simulink model "PMSM_FOC_Encoder_ST"  (R2013b)
settings: Solver=FixedStepDiscrete  StartTime=0.0  StopTime=0.8  FixedStep=1/10000  RelTol=1e-3
PostLoadFcn:
  | PMSM_Params
undefined symbols (not defined in the file or in its folder): Params, PC10, PC11, uart4, usart3
libraries: ADC_Lib x5, GPIO_Lib x5, TIMERS_Lib x2, USART_Lib x1
settings Model: Creator=Alex  LastModifiedBy=reynaudp
settings OptimizationCC: ExpressionDepthLimit=2147483647  OptimizeModelRefInitCode=on  LifeSpan=1
settings DebuggingCC: StateNameClashWarn=warning
settings HardwareCC: ProdLargestAtomicInteger=Integer  ProdLargestAtomicFloat=Float  ProdIntDivRoundTo=Zero  ProdEndianess=LittleEndian  ProdHWDeviceType=STMicroelectronics->STM32F4xx 32-bit Cortex-M4  TargetLargestAtomicInteger=Integer  TargetLargestAtomicFloat=Float  TargetIntDivRoundTo=Zero  TargetEndianess=LittleEndian  TargetHWDeviceType=STMicroelectronics->STM32F4xx 32-bit Cortex-M4
settings RTWCC: SystemTargetFile=stm32F4xx.tlc  TemplateMakefile=stm32F4xx.tmf  Description=stm32F4xx (Embedded Target)  GenerateReport=on  ProcessScript=stm32F4xx_make_rtw_hook  IncludeHyperlinkInReport=on  LaunchReport=on  GenerateCodeReplacementReport=on
settings CodeAppCC: IgnoreCustomStorageClasses=off  MaxIdLength=64  CustomSymbolStrType=$N$R$M  InternalIdentifier=Classic
settings STFCustomTargetCC: ParMdlRefBuildCompliant=on  IncludeMdlTerminateFcn=off  CombineOutputUpdateFcns=on  ERTCustomFileBanners=on  SupportContinuousTime=off  SupportNonInlinedSFcns=off  MATLABClassNameForMDSCustomization=Simulink.SoftwareTarget.ERTCustomization  GRTInterface=off  SystemTargetFile=stm32F4xx.tlc
settings ERTTargetCC: CodeReplacementLibrary=ANSI_C  CompOptLevelCompliant=off  ConcurrentExecutionCompliant=off  IncludeMdlTerminateFcn=off  ERTFirstTimeCompliant=off  ModelStepFunctionPrototypeControlCompliant=off  CPPClassGenCompliant=off  InlinedParameterPlacement=NonHierarchical  ERTSrcFileBannerTemplate=sourceFileTemplate.cgt  ERTHdrFileBannerTemplate=sourceFileTemplate.cgt  ERTDataSrcFileTemplate=sourceFileTemplate.cgt  ERTDataHdrFileTemplate=sourceFileTemplate.cgt  ERTCustomFileTemplate=customRoutineProcess.tlc

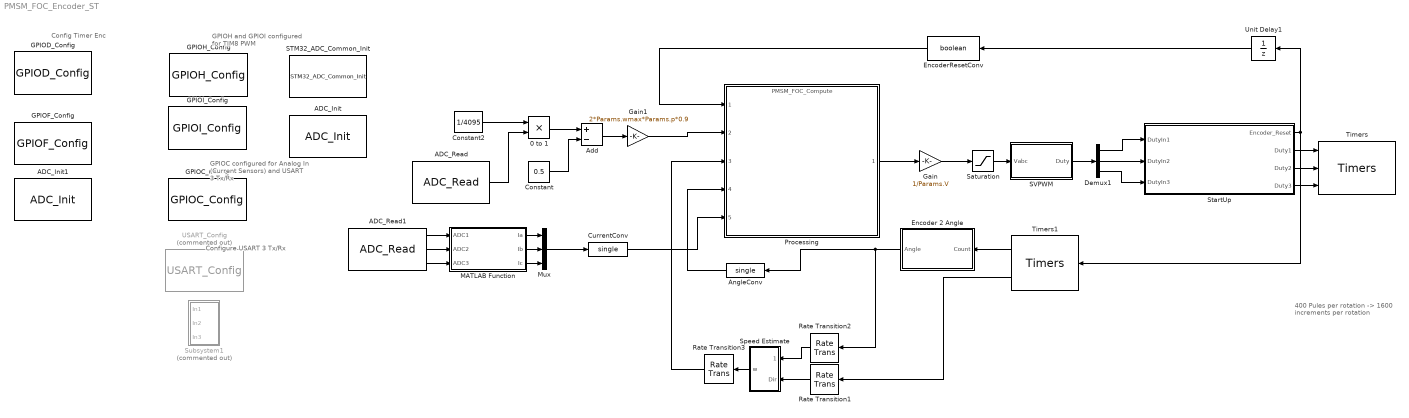
== system PMSM_FOC_Encoder_ST ==
  note: Config Timer Enc
  note: 400 Pules per rotation -> 1600 increments per rotation
  note: Configure USART 3 Tx/Rx
  note: GPIOC configured for Analog In (Current Sensors)
      | and  USART 3 Tx/Rx
  note: GPIOH and GPIOI configured for TIM8 PWM
  0 to 1 : Product  RndMeth=Zero
  ADC_Init : ADC_Lib/ADC_Init  ADC_Name=ADC1  ADC_Type=Regular  ADC_Default=off  ADC_Offset=0  ADC_Resolution=ADC_Resolution_12b  ADC_ScanConvMode=Multichannels  ADC_ContinuousConvMode=on  ADC_ExtTrigPol=ADC_ExternalTrigConvEdge_Rising  ADC_ExtTrigInjPol=ADC_ExternalTrigInjecConvEdge_None  ADC_ExtTrig=ADC_ExternalTrigConv_T8_TRGO  ADC_ExtTrigInj=ADC_ExternalTrigInjecConv_T1_CC4  ADC_DataAlign=ADC_DataAlign_Right  ADC_NbConv=3  ADC_DMA_channel=DMA_Channel_0  ADC_DMA_stream=DMA2_Stream0  ADC_Watchdog_Enable=off  ADC_Watchdog_Command=ADC_AnalogWatchdog_None  ADC_Watchdog_NumChan=0  ADC_Watchdog_HighThreshold=4095  ADC_Watchdog_lowThreshold=0  ADC_Ch0=off  ADC_Ch0T=Regular  ADC_Ch0L=PA0  ADC_Ch1=off  ADC_Ch1T=Regular  ADC_Ch1L=PA1  ADC_Ch2=off  ADC_Ch2T=Regular  ADC_Ch2L=PA2  ADC_Ch3=off  ADC_Ch3T=Regular  ADC_Ch3L=PA3  ADC_Ch4=off  ADC_Ch4T=Regular  ADC_Ch4L=PA4  ADC_Ch5=off  ADC_Ch5T=Regular  ADC_Ch5L=PA5  ADC_Ch6=off  ADC_Ch6T=Regular  ADC_Ch6L=PA6  ADC_Ch7=off  ADC_Ch7T=Regular  ADC_Ch7L=PA7  ADC_Ch8=off  ADC_Ch8T=Regular  ADC_Ch8L=PB0  ADC_Ch9=off  ADC_Ch9T=Regular  ADC_Ch9L=PB1  ADC_Ch10=off  ADC_Ch10T=Regular  ADC_Ch10L=PC0  ADC_Ch11=on  ADC_Ch11T=Regular  ADC_Ch11L=PC1  ADC_Ch12=on  ADC_Ch12T=Regular  ADC_Ch12L=PC2  ADC_Ch13=on  ADC_Ch13T=Regular  ADC_Ch13L=PC3  ADC_Ch14=off  ADC_Ch14T=Regular  ADC_Ch14L=PC4  ADC_Ch15=off  ADC_Ch15T=Regular  ADC_Ch15L=PC5  ADC_Ch16=off  ADC_Ch16T=Regular  ADC_Ch16L=Temp.Sensor  ADC_Ch17=off  ADC_Ch17T=Regular  ADC_Ch17L=Vrefint  ADC_Ch18=off  ADC_Ch18T=Regular  ADC_Ch18L=Vbat
  ADC_Init1 : ADC_Lib/ADC_Init  ADC_Name=ADC3  ADC_Type=Regular  ADC_Default=off  ADC_Offset=0  ADC_Resolution=ADC_Resolution_12b  ADC_ScanConvMode=One_channel  ADC_ContinuousConvMode=on  ADC_ExtTrigPol=ADC_ExternalTrigConvEdge_None  ADC_ExtTrigInjPol=ADC_ExternalTrigInjecConvEdge_None  ADC_ExtTrig=ADC_ExternalTrigConv_T1_CC1  ADC_ExtTrigInj=ADC_ExternalTrigInjecConv_T1_CC4  ADC_DataAlign=ADC_DataAlign_Right  ADC_NbConv=1  ADC_DMA_channel=not_used  ADC_DMA_stream=not_used  ADC_Watchdog_Enable=off  ADC_Watchdog_Command=ADC_AnalogWatchdog_None  ADC_Watchdog_NumChan=0  ADC_Watchdog_HighThreshold=4095  ADC_Watchdog_lowThreshold=0  ADC_Ch0=off  ADC_Ch0T=Regular  ADC_Ch0L=PA0  ADC_Ch1=off  ADC_Ch1T=Regular  ADC_Ch1L=PA1  ADC_Ch2=off  ADC_Ch2T=Regular  ADC_Ch2L=PA2  ADC_Ch3=off  ADC_Ch3T=Regular  ADC_Ch3L=PA3  ADC_Ch4=off  ADC_Ch4T=Regular  ADC_Ch4L=PF6  ADC_Ch5=off  ADC_Ch5T=Regular  ADC_Ch5L=PF7  ADC_Ch6=off  ADC_Ch6T=Regular  ADC_Ch6L=PF8  ADC_Ch7=on  ADC_Ch7T=Regular  ADC_Ch7L=PF9  ADC_Ch8=off  ADC_Ch8T=Regular  ADC_Ch8L=PF10  ADC_Ch9=off  ADC_Ch9T=Regular  ADC_Ch9L=PF3  ADC_Ch10=off  ADC_Ch10T=Regular  ADC_Ch10L=PC0  ADC_Ch11=off  ADC_Ch11T=Regular  ADC_Ch11L=PC1  ADC_Ch12=off  ADC_Ch12T=Regular  ADC_Ch12L=PC2  ADC_Ch13=off  ADC_Ch13T=Regular  ADC_Ch13L=PC3  ADC_Ch14=off  ADC_Ch14T=Regular  ADC_Ch14L=PF4  ADC_Ch15=off  ADC_Ch15T=Regular  ADC_Ch15L=PF5  ADC_Ch16=off  ADC_Ch16T=Regular  ADC_Ch17=off  ADC_Ch17T=Regular  ADC_Ch18=off  ADC_Ch18T=Regular
  ADC_Read : ADC_Lib/ADC_Read  ADC_Name=ADC3  ADC_Ch0=off  ADC_Ch1=off  ADC_Ch2=off  ADC_Ch3=off  ADC_Ch4=off  ADC_Ch5=off  ADC_Ch6=off  ADC_Ch7=on  ADC_Ch8=off  ADC_Ch9=off  ADC_Ch10=off  ADC_Ch11=off  ADC_Ch12=off  ADC_Ch13=off  ADC_Ch14=off  ADC_Ch15=off  ADC_Ch16=off  ADC_Ch17=off  ADC_Ch18=off
  ADC_Read1 : ADC_Lib/ADC_Read  ADC_Name=ADC1  ADC_Ch0=off  ADC_Ch1=off  ADC_Ch2=off  ADC_Ch3=off  ADC_Ch4=off  ADC_Ch5=off  ADC_Ch6=off  ADC_Ch7=off  ADC_Ch8=off  ADC_Ch9=off  ADC_Ch10=off  ADC_Ch11=on  ADC_Ch12=on  ADC_Ch13=on  ADC_Ch14=off  ADC_Ch15=off  ADC_Ch16=off  ADC_Ch17=off  ADC_Ch18=off
  Add : Sum  Inputs=+-
  AngleConv : DataTypeConversion  OutDataTypeStr=single
  Constant : Constant  Value=0.5
  Constant2 : Constant  Value=1/4095
  CurrentConv : DataTypeConversion  OutDataTypeStr=single
  Demux1 : Demux  Outputs=3
  Encoder 2 Angle : MATLAB Function  TreatAsAtomicUnit=on
      settings: MinAlgLoopOccurrences=on
  EncoderResetConv : DataTypeConversion  OutDataTypeStr=boolean
  GPIOC_Config : GPIO_Lib/GPIOC_Config  Pin0_Use=off  Pin1_Use=on  Pin2_Use=on  Pin3_Use=on  Pin4_Use=off  Pin5_Use=off  Pin6_Use=off  Pin7_Use=on  Pin8_Use=off  Pin9_Use=off  Pin10_Use=on  Pin11_Use=on  Pin12_Use=off  Pin13_Use=off  Pin14_Use=off  Pin15_Use=off  Pin0_Speed=GPIO_Speed_2MHz  Pin1_Speed=GPIO_Speed_25MHz  Pin2_Speed=GPIO_Speed_25MHz  Pin3_Speed=GPIO_Speed_25MHz  Pin4_Speed=GPIO_Speed_2MHz  Pin5_Speed=GPIO_Speed_2MHz  Pin6_Speed=GPIO_Speed_2MHz  Pin7_Speed=GPIO_Speed_50MHz  Pin8_Speed=GPIO_Speed_2MHz  Pin9_Speed=GPIO_Speed_2MHz  Pin10_Speed=GPIO_Speed_2MHz  Pin11_Speed=GPIO_Speed_2MHz  Pin12_Speed=GPIO_Speed_2MHz  Pin13_Speed=GPIO_Speed_2MHz  Pin14_Speed=GPIO_Speed_2MHz  Pin15_Speed=GPIO_Speed_2MHz  Pin0_Mode=GPIO_Mode_OUT  Pin1_Mode=GPIO_Mode_AN  Pin2_Mode=GPIO_Mode_AN  Pin3_Mode=GPIO_Mode_AN  Pin4_Mode=GPIO_Mode_OUT  Pin5_Mode=GPIO_Mode_OUT  Pin6_Mode=GPIO_Mode_OUT  Pin7_Mode=GPIO_Mode_OUT  Pin8_Mode=GPIO_Mode_OUT  Pin9_Mode=GPIO_Mode_OUT  Pin10_Mode=GPIO_Mode_AF  Pin11_Mode=GPIO_Mode_AF  Pin12_Mode=GPIO_Mode_OUT  Pin13_Mode=GPIO_Mode_OUT  Pin14_Mode=GPIO_Mode_OUT  Pin15_Mode=GPIO_Mode_OUT  Pin0_Type=GPIO_OType_PP  Pin1_Type=GPIO_OType_PP  Pin2_Type=GPIO_OType_PP  Pin3_Type=GPIO_OType_PP  Pin4_Type=GPIO_OType_PP  Pin5_Type=GPIO_OType_PP  Pin6_Type=GPIO_OType_PP  Pin7_Type=GPIO_OType_PP  Pin8_Type=GPIO_OType_PP  Pin9_Type=GPIO_OType_PP  Pin10_Type=GPIO_OType_PP  Pin11_Type=GPIO_OType_PP  Pin12_Type=GPIO_OType_PP  Pin13_Type=GPIO_OType_PP  Pin14_Type=GPIO_OType_PP  Pin15_Type=GPIO_OType_PP  Pin0_PuPd=GPIO_PuPd_NOPULL  Pin1_PuPd=GPIO_PuPd_NOPULL  Pin2_PuPd=GPIO_PuPd_NOPULL  Pin3_PuPd=GPIO_PuPd_NOPULL  Pin4_PuPd=GPIO_PuPd_NOPULL  Pin5_PuPd=GPIO_PuPd_NOPULL  Pin6_PuPd=GPIO_PuPd_NOPULL  Pin7_PuPd=GPIO_PuPd_NOPULL  Pin8_PuPd=GPIO_PuPd_NOPULL  Pin9_PuPd=GPIO_PuPd_NOPULL  Pin10_PuPd=GPIO_PuPd_NOPULL  Pin11_PuPd=GPIO_PuPd_NOPULL  Pin12_PuPd=GPIO_PuPd_NOPULL  Pin13_PuPd=GPIO_PuPd_NOPULL  Pin14_PuPd=GPIO_PuPd_NOPULL  Pin15_PuPd=GPIO_PuPd_NOPULL  Pin0_AF=GPIO_AF_OTG_HS  Pin1_AF=GPIO_AF_ETH  Pin2_AF=GPIO_AF_SPI2  Pin3_AF=GPIO_AF_SPI2  Pin4_AF=GPIO_AF_ETH  Pin5_AF=GPIO_AF_EVENTOUT  Pin6_AF=GPIO_AF_TIM3  Pin7_AF=GPIO_AF_TIM3  Pin8_AF=GPIO_AF_TIM3  Pin9_AF=GPIO_AF_MCO  Pin10_AF=GPIO_AF_USART3  Pin11_AF=GPIO_AF_USART3  Pin12_AF=GPIO_AF_USART3  Pin0_Set=off  Pin1_Set=off  Pin2_Set=off  Pin3_Set=off  Pin4_Set=off  Pin5_Set=off  Pin6_Set=off  Pin7_Set=off  Pin8_Set=off  Pin9_Set=off  Pin10_Set=off  Pin11_Set=off  Pin12_Set=off  Pin13_Set=off  Pin14_Set=off  Pin15_Set=off
  GPIOD_Config : GPIO_Lib/GPIOD_Config  Pin0_Use=off  Pin1_Use=off  Pin2_Use=off  Pin3_Use=off  Pin4_Use=off  Pin5_Use=off  Pin6_Use=off  Pin7_Use=off  Pin8_Use=off  Pin9_Use=off  Pin10_Use=off  Pin11_Use=off  Pin12_Use=on  Pin13_Use=on  Pin14_Use=off  Pin15_Use=off  Pin0_Speed=GPIO_Speed_2MHz  Pin1_Speed=GPIO_Speed_2MHz  Pin2_Speed=GPIO_Speed_2MHz  Pin3_Speed=GPIO_Speed_2MHz  Pin4_Speed=GPIO_Speed_2MHz  Pin5_Speed=GPIO_Speed_2MHz  Pin6_Speed=GPIO_Speed_2MHz  Pin7_Speed=GPIO_Speed_2MHz  Pin8_Speed=GPIO_Speed_2MHz  Pin9_Speed=GPIO_Speed_2MHz  Pin10_Speed=GPIO_Speed_2MHz  Pin11_Speed=GPIO_Speed_2MHz  Pin12_Speed=GPIO_Speed_50MHz  Pin13_Speed=GPIO_Speed_50MHz  Pin14_Speed=GPIO_Speed_2MHz  Pin15_Speed=GPIO_Speed_2MHz  Pin0_Mode=GPIO_Mode_OUT  Pin1_Mode=GPIO_Mode_OUT  Pin2_Mode=GPIO_Mode_OUT  Pin3_Mode=GPIO_Mode_OUT  Pin4_Mode=GPIO_Mode_OUT  Pin5_Mode=GPIO_Mode_OUT  Pin6_Mode=GPIO_Mode_OUT  Pin7_Mode=GPIO_Mode_OUT  Pin8_Mode=GPIO_Mode_OUT  Pin9_Mode=GPIO_Mode_OUT  Pin10_Mode=GPIO_Mode_OUT  Pin11_Mode=GPIO_Mode_OUT  Pin12_Mode=GPIO_Mode_AF  Pin13_Mode=GPIO_Mode_AF  Pin14_Mode=GPIO_Mode_OUT  Pin15_Mode=GPIO_Mode_OUT  Pin0_Type=GPIO_OType_PP  Pin1_Type=GPIO_OType_PP  Pin2_Type=GPIO_OType_PP  Pin3_Type=GPIO_OType_PP  Pin4_Type=GPIO_OType_PP  Pin5_Type=GPIO_OType_PP  Pin6_Type=GPIO_OType_PP  Pin7_Type=GPIO_OType_PP  Pin8_Type=GPIO_OType_PP  Pin9_Type=GPIO_OType_PP  Pin10_Type=GPIO_OType_PP  Pin11_Type=GPIO_OType_PP  Pin12_Type=GPIO_OType_PP  Pin13_Type=GPIO_OType_PP  Pin14_Type=GPIO_OType_PP  Pin15_Type=GPIO_OType_PP  Pin0_PuPd=GPIO_PuPd_NOPULL  Pin1_PuPd=GPIO_PuPd_NOPULL  Pin2_PuPd=GPIO_PuPd_NOPULL  Pin3_PuPd=GPIO_PuPd_NOPULL  Pin4_PuPd=GPIO_PuPd_NOPULL  Pin5_PuPd=GPIO_PuPd_NOPULL  Pin6_PuPd=GPIO_PuPd_NOPULL  Pin7_PuPd=GPIO_PuPd_NOPULL  Pin8_PuPd=GPIO_PuPd_NOPULL  Pin9_PuPd=GPIO_PuPd_NOPULL  Pin10_PuPd=GPIO_PuPd_NOPULL  Pin11_PuPd=GPIO_PuPd_NOPULL  Pin12_PuPd=GPIO_PuPd_NOPULL  Pin13_PuPd=GPIO_PuPd_NOPULL  Pin14_PuPd=GPIO_PuPd_NOPULL  Pin15_PuPd=GPIO_PuPd_NOPULL  Pin0_AF=GPIO_AF_CAN1  Pin1_AF=GPIO_AF_CAN1  Pin2_AF=GPIO_AF_TIM3  Pin3_AF=GPIO_AF_USART2  Pin4_AF=GPIO_AF_USART2  Pin5_AF=GPIO_AF_EVENTOUT  Pin6_AF=GPIO_AF_USART2  Pin7_AF=GPIO_AF_USART2  Pin8_AF=GPIO_AF_USART3  Pin9_AF=GPIO_AF_USART3  Pin10_AF=GPIO_AF_USART3  Pin11_AF=GPIO_AF_USART3  Pin12_AF=GPIO_AF_TIM4  Pin13_AF=GPIO_AF_TIM4  Pin14_AF=GPIO_AF_TIM4  Pin15_AF=GPIO_AF_EVENTOUT  Pin0_Set=off  Pin1_Set=off  Pin2_Set=off  Pin3_Set=off  Pin4_Set=off  Pin5_Set=off  Pin6_Set=off  Pin7_Set=off  Pin8_Set=off  Pin9_Set=off  Pin10_Set=off  Pin11_Set=off  Pin12_Set=off  Pin13_Set=off  Pin14_Set=off  Pin15_Set=off
  GPIOF_Config : GPIO_Lib/GPIOF_Config  Pin0_Use=off  Pin1_Use=off  Pin2_Use=off  Pin3_Use=off  Pin4_Use=off  Pin5_Use=off  Pin6_Use=off  Pin7_Use=off  Pin8_Use=off  Pin9_Use=on  Pin10_Use=off  Pin11_Use=off  Pin12_Use=off  Pin13_Use=off  Pin14_Use=off  Pin15_Use=off  Pin0_Speed=GPIO_Speed_2MHz  Pin1_Speed=GPIO_Speed_2MHz  Pin2_Speed=GPIO_Speed_2MHz  Pin3_Speed=GPIO_Speed_2MHz  Pin4_Speed=GPIO_Speed_2MHz  Pin5_Speed=GPIO_Speed_2MHz  Pin6_Speed=GPIO_Speed_2MHz  Pin7_Speed=GPIO_Speed_2MHz  Pin8_Speed=GPIO_Speed_2MHz  Pin9_Speed=GPIO_Speed_50MHz  Pin10_Speed=GPIO_Speed_2MHz  Pin11_Speed=GPIO_Speed_2MHz  Pin12_Speed=GPIO_Speed_2MHz  Pin13_Speed=GPIO_Speed_2MHz  Pin14_Speed=GPIO_Speed_2MHz  Pin15_Speed=GPIO_Speed_2MHz  Pin0_Mode=GPIO_Mode_OUT  Pin1_Mode=GPIO_Mode_OUT  Pin2_Mode=GPIO_Mode_OUT  Pin3_Mode=GPIO_Mode_OUT  Pin4_Mode=GPIO_Mode_OUT  Pin5_Mode=GPIO_Mode_OUT  Pin6_Mode=GPIO_Mode_OUT  Pin7_Mode=GPIO_Mode_OUT  Pin8_Mode=GPIO_Mode_OUT  Pin9_Mode=GPIO_Mode_AN  Pin10_Mode=GPIO_Mode_OUT  Pin11_Mode=GPIO_Mode_OUT  Pin12_Mode=GPIO_Mode_OUT  Pin13_Mode=GPIO_Mode_OUT  Pin14_Mode=GPIO_Mode_OUT  Pin15_Mode=GPIO_Mode_OUT  Pin0_Type=GPIO_OType_PP  Pin1_Type=GPIO_OType_PP  Pin2_Type=GPIO_OType_PP  Pin3_Type=GPIO_OType_PP  Pin4_Type=GPIO_OType_PP  Pin5_Type=GPIO_OType_PP  Pin6_Type=GPIO_OType_PP  Pin7_Type=GPIO_OType_PP  Pin8_Type=GPIO_OType_PP  Pin9_Type=GPIO_OType_PP  Pin10_Type=GPIO_OType_PP  Pin11_Type=GPIO_OType_PP  Pin12_Type=GPIO_OType_PP  Pin13_Type=GPIO_OType_PP  Pin14_Type=GPIO_OType_PP  Pin15_Type=GPIO_OType_PP  Pin0_PuPd=GPIO_PuPd_NOPULL  Pin1_PuPd=GPIO_PuPd_NOPULL  Pin2_PuPd=GPIO_PuPd_NOPULL  Pin3_PuPd=GPIO_PuPd_NOPULL  Pin4_PuPd=GPIO_PuPd_NOPULL  Pin5_PuPd=GPIO_PuPd_NOPULL  Pin6_PuPd=GPIO_PuPd_NOPULL  Pin7_PuPd=GPIO_PuPd_NOPULL  Pin8_PuPd=GPIO_PuPd_NOPULL  Pin9_PuPd=GPIO_PuPd_NOPULL  Pin10_PuPd=GPIO_PuPd_NOPULL  Pin11_PuPd=GPIO_PuPd_NOPULL  Pin12_PuPd=GPIO_PuPd_NOPULL  Pin13_PuPd=GPIO_PuPd_NOPULL  Pin14_PuPd=GPIO_PuPd_NOPULL  Pin15_PuPd=GPIO_PuPd_NOPULL  Pin0_AF=GPIO_AF_I2C2  Pin1_AF=GPIO_AF_FSMC  Pin2_AF=GPIO_AF_I2C2  Pin3_AF=GPIO_AF_FSMC  Pin4_AF=GPIO_AF_FSMC  Pin5_AF=GPIO_AF_EVENTOUT  Pin6_AF=GPIO_AF_TIM10  Pin7_AF=GPIO_AF_TIM11  Pin8_AF=GPIO_AF_TIM13  Pin9_AF=GPIO_AF_TIM14  Pin10_AF=GPIO_AF_FSMC  Pin11_AF=GPIO_AF_DCMI  Pin12_AF=GPIO_AF_FSMC  Pin13_AF=GPIO_AF_FSMC  Pin14_AF=GPIO_AF_FSMC  Pin15_AF=GPIO_AF_EVENTOUT  Pin0_Set=off  Pin1_Set=off  Pin2_Set=off  Pin3_Set=off  Pin4_Set=off  Pin5_Set=off  Pin6_Set=off  Pin7_Set=off  Pin8_Set=off  Pin9_Set=off  Pin10_Set=off  Pin11_Set=off  Pin12_Set=off  Pin13_Set=off  Pin14_Set=off  Pin15_Set=off
  GPIOH_Config : GPIO_Lib/GPIOH_Config  Pin0_Use=off  Pin1_Use=off  Pin2_Use=off  Pin3_Use=off  Pin4_Use=off  Pin5_Use=off  Pin6_Use=off  Pin7_Use=off  Pin8_Use=off  Pin9_Use=off  Pin10_Use=off  Pin11_Use=off  Pin12_Use=off  Pin13_Use=on  Pin14_Use=on  Pin15_Use=on  Pin0_Speed=GPIO_Speed_2MHz  Pin1_Speed=GPIO_Speed_2MHz  Pin2_Speed=GPIO_Speed_2MHz  Pin3_Speed=GPIO_Speed_2MHz  Pin4_Speed=GPIO_Speed_2MHz  Pin5_Speed=GPIO_Speed_2MHz  Pin6_Speed=GPIO_Speed_2MHz  Pin7_Speed=GPIO_Speed_2MHz  Pin8_Speed=GPIO_Speed_2MHz  Pin9_Speed=GPIO_Speed_2MHz  Pin10_Speed=GPIO_Speed_2MHz  Pin11_Speed=GPIO_Speed_2MHz  Pin12_Speed=GPIO_Speed_2MHz  Pin13_Speed=GPIO_Speed_50MHz  Pin14_Speed=GPIO_Speed_50MHz  Pin15_Speed=GPIO_Speed_50MHz  Pin0_Mode=GPIO_Mode_OUT  Pin1_Mode=GPIO_Mode_OUT  Pin2_Mode=GPIO_Mode_OUT  Pin3_Mode=GPIO_Mode_OUT  Pin4_Mode=GPIO_Mode_OUT  Pin5_Mode=GPIO_Mode_OUT  Pin6_Mode=GPIO_Mode_OUT  Pin7_Mode=GPIO_Mode_OUT  Pin8_Mode=GPIO_Mode_OUT  Pin9_Mode=GPIO_Mode_OUT  Pin10_Mode=GPIO_Mode_OUT  Pin11_Mode=GPIO_Mode_OUT  Pin12_Mode=GPIO_Mode_OUT  Pin13_Mode=GPIO_Mode_AF  Pin14_Mode=GPIO_Mode_AF  Pin15_Mode=GPIO_Mode_AF  Pin0_Type=GPIO_OType_PP  Pin1_Type=GPIO_OType_PP  Pin2_Type=GPIO_OType_PP  Pin3_Type=GPIO_OType_PP  Pin4_Type=GPIO_OType_PP  Pin5_Type=GPIO_OType_PP  Pin6_Type=GPIO_OType_PP  Pin7_Type=GPIO_OType_PP  Pin8_Type=GPIO_OType_PP  Pin9_Type=GPIO_OType_PP  Pin10_Type=GPIO_OType_PP  Pin11_Type=GPIO_OType_PP  Pin12_Type=GPIO_OType_PP  Pin13_Type=GPIO_OType_PP  Pin14_Type=GPIO_OType_PP  Pin15_Type=GPIO_OType_PP  Pin0_PuPd=GPIO_PuPd_NOPULL  Pin1_PuPd=GPIO_PuPd_NOPULL  Pin2_PuPd=GPIO_PuPd_NOPULL  Pin3_PuPd=GPIO_PuPd_NOPULL  Pin4_PuPd=GPIO_PuPd_NOPULL  Pin5_PuPd=GPIO_PuPd_NOPULL  Pin6_PuPd=GPIO_PuPd_NOPULL  Pin7_PuPd=GPIO_PuPd_NOPULL  Pin8_PuPd=GPIO_PuPd_NOPULL  Pin9_PuPd=GPIO_PuPd_NOPULL  Pin10_PuPd=GPIO_PuPd_NOPULL  Pin11_PuPd=GPIO_PuPd_NOPULL  Pin12_PuPd=GPIO_PuPd_NOPULL  Pin13_PuPd=GPIO_PuPd_NOPULL  Pin14_PuPd=GPIO_PuPd_NOPULL  Pin15_PuPd=GPIO_PuPd_NOPULL  Pin2_AF=GPIO_AF_ETH  Pin3_AF=GPIO_AF_ETH  Pin4_AF=GPIO_AF_I2C2  Pin5_AF=GPIO_AF_EVENTOUT  Pin6_AF=GPIO_AF_I2C2  Pin7_AF=GPIO_AF_I2C3  Pin8_AF=GPIO_AF_I2C3  Pin9_AF=GPIO_AF_I2C3  Pin10_AF=GPIO_AF_TIM5  Pin11_AF=GPIO_AF_TIM5  Pin12_AF=GPIO_AF_TIM5  Pin13_AF=GPIO_AF_TIM8  Pin14_AF=GPIO_AF_TIM8  Pin15_AF=GPIO_AF_TIM8  Pin0_Set=off  Pin1_Set=off  Pin2_Set=off  Pin3_Set=off  Pin4_Set=off  Pin5_Set=off  Pin6_Set=off  Pin7_Set=off  Pin8_Set=off  Pin9_Set=off  Pin10_Set=off  Pin11_Set=off  Pin12_Set=off  Pin13_Set=off  Pin14_Set=off  Pin15_Set=off
  GPIOI_Config : GPIO_Lib/GPIOI_Config  Pin0_Use=off  Pin1_Use=off  Pin2_Use=off  Pin3_Use=off  Pin4_Use=off  Pin5_Use=on  Pin6_Use=on  Pin7_Use=on  Pin8_Use=off  Pin9_Use=off  Pin10_Use=off  Pin11_Use=off  Pin0_Speed=GPIO_Speed_2MHz  Pin1_Speed=GPIO_Speed_2MHz  Pin2_Speed=GPIO_Speed_2MHz  Pin3_Speed=GPIO_Speed_2MHz  Pin4_Speed=GPIO_Speed_2MHz  Pin5_Speed=GPIO_Speed_50MHz  Pin6_Speed=GPIO_Speed_50MHz  Pin7_Speed=GPIO_Speed_50MHz  Pin8_Speed=GPIO_Speed_2MHz  Pin9_Speed=GPIO_Speed_2MHz  Pin10_Speed=GPIO_Speed_2MHz  Pin11_Speed=GPIO_Speed_2MHz  Pin0_Mode=GPIO_Mode_OUT  Pin1_Mode=GPIO_Mode_OUT  Pin2_Mode=GPIO_Mode_OUT  Pin3_Mode=GPIO_Mode_OUT  Pin4_Mode=GPIO_Mode_OUT  Pin5_Mode=GPIO_Mode_AF  Pin6_Mode=GPIO_Mode_AF  Pin7_Mode=GPIO_Mode_AF  Pin8_Mode=GPIO_Mode_OUT  Pin9_Mode=GPIO_Mode_OUT  Pin10_Mode=GPIO_Mode_OUT  Pin11_Mode=GPIO_Mode_OUT  Pin0_Type=GPIO_OType_PP  Pin1_Type=GPIO_OType_PP  Pin2_Type=GPIO_OType_PP  Pin3_Type=GPIO_OType_PP  Pin4_Type=GPIO_OType_PP  Pin5_Type=GPIO_OType_PP  Pin6_Type=GPIO_OType_PP  Pin7_Type=GPIO_OType_PP  Pin8_Type=GPIO_OType_PP  Pin9_Type=GPIO_OType_PP  Pin10_Type=GPIO_OType_PP  Pin11_Type=GPIO_OType_PP  Pin0_PuPd=GPIO_PuPd_NOPULL  Pin1_PuPd=GPIO_PuPd_NOPULL  Pin2_PuPd=GPIO_PuPd_NOPULL  Pin3_PuPd=GPIO_PuPd_NOPULL  Pin4_PuPd=GPIO_PuPd_NOPULL  Pin5_PuPd=GPIO_PuPd_NOPULL  Pin6_PuPd=GPIO_PuPd_NOPULL  Pin7_PuPd=GPIO_PuPd_NOPULL  Pin8_PuPd=GPIO_PuPd_NOPULL  Pin9_PuPd=GPIO_PuPd_NOPULL  Pin10_PuPd=GPIO_PuPd_NOPULL  Pin11_PuPd=GPIO_PuPd_NOPULL  Pin0_AF=GPIO_AF_TIM5  Pin1_AF=GPIO_AF_SPI2  Pin2_AF=GPIO_AF_TIM8  Pin3_AF=GPIO_AF_TIM8  Pin4_AF=GPIO_AF_TIM8  Pin5_AF=GPIO_AF_TIM8  Pin6_AF=GPIO_AF_TIM8  Pin7_AF=GPIO_AF_TIM8  Pin9_AF=GPIO_AF_CAN1  Pin10_AF=GPIO_AF_ETH  Pin11_AF=GPIO_AF_OTG_HS  Pin0_Set=off  Pin1_Set=off  Pin2_Set=off  Pin3_Set=off  Pin4_Set=off  Pin5_Set=off  Pin6_Set=off  Pin7_Set=off  Pin8_Set=off  Pin9_Set=off  Pin10_Set=off  Pin11_Set=off
  Gain : Gain  Gain=1/Params.V
  Gain1 : Gain  Gain=2*Params.wmax*Params.p*0.9
  MATLAB Function : MATLAB Function  TreatAsAtomicUnit=on
  Mux : Mux  Inputs=3
  Processing : ModelReference  ModelNameDialog=PMSM_FOC_Compute.slx  SimulationMode=Normal  ModelReferenceVersion=1.77  CopyOfModelName=PMSM_FOC_Compute.slx  DefaultDataLogging=on
  Rate Transition1 : RateTransition
  Rate Transition2 : RateTransition
  Rate Transition3 : RateTransition
  STM32_ADC_Common_Init : ADC_Lib/STM32_ADC_Common_Init  ADC_Mode=ADC_Mode_Independent  ADC_Prescaler=ADC_Prescaler_Div2  ADC_DMAAccessMode=ADC_DMAAccessMode_Disabled  ADC_TwoSamplingDelay=ADC_TwoSamplingDelay_5Cycles
  SVPWM : MATLAB Function  TreatAsAtomicUnit=on
  Saturation : Saturate  UpperLimit=1  LowerLimit=-1
  Speed Estimate : Subsystem  TreatAsAtomicUnit=on  SystemSampleTime=1/100
  StartUp : Stateflow chart  TreatAsAtomicUnit=on
      settings: MinAlgLoopOccurrences=on
  Subsystem1 : Subsystem  Commented=on
  Timers : TIMERS_Lib/Timers  Timer_name=TIM8  Timer_clock=20000000  Timer_mode=TIM_CounterMode_CenterAligned2  Timer_inout=Output_PWM  Variable_frequency=off  Output_frequency=40000  Encoder_mode=TIM_EncoderMode_TI12  Encoder_auto_reload=0  TRGO_source=TIM_TRGOSource_Enable  Repetition_counter=0  CH1_enable=on  CH1_type=Output  CH1_int=off  CH1_variable_duty=on  CH1_output_duty=50  CH1_output_polarity=TIM_OCPolarity_Low  CH1_output_comp_state=on  CH1_output_comp_polarity=TIM_OCNPolarity_Low  CH1_output_idle=TIM_OCIdleState_Set  CH1_output_comp_idle=TIM_OCNIdleState_Reset  CH1_input_polarity=TIM_ICPolarity_Rising  CH1_input_prescaler=TIM_ICPSC_DIV1  CH1_input_filter=0  CH1_input_it=No_interrupt  Encoder_TI1_polarity=TIM_ICPolarity_Falling  CH2_enable=on  CH2_type=Output  CH2_int=off  CH2_variable_duty=on  CH2_output_duty=50  CH2_output_polarity=TIM_OCPolarity_Low  CH2_output_comp_state=on  CH2_output_comp_polarity=TIM_OCNPolarity_Low  CH2_output_idle=TIM_OCIdleState_Set  CH2_output_comp_idle=TIM_OCNIdleState_Reset  CH2_input_polarity=TIM_ICPolarity_Rising  CH2_input_prescaler=TIM_ICPSC_DIV1  CH2_input_filter=0  CH2_input_it=No_interrupt  Encoder_TI2_polarity=TIM_ICPolarity_Falling  CH3_enable=on  CH3_type=Output  CH3_int=off  CH3_variable_duty=on  CH3_output_duty=50  CH3_output_polarity=TIM_OCPolarity_Low  CH3_output_comp_state=on  CH3_output_comp_polarity=TIM_OCNPolarity_Low  CH3_output_idle=TIM_OCIdleState_Set  CH3_output_comp_idle=TIM_OCNIdleState_Reset  CH3_input_polarity=TIM_ICPolarity_Rising  CH3_input_prescaler=TIM_ICPSC_DIV1  CH3_input_filter=0  CH3_input_it=No_interrupt
  Timers1 : TIMERS_Lib/Timers  Timer_name=TIM4  Timer_clock=21000000  Timer_mode=TIM_CounterMode_Up  Timer_inout=Encoder  Variable_frequency=off  Output_frequency=100000  Encoder_mode=TIM_EncoderMode_TI12  Encoder_auto_reload=1600-1  TRGO_source=not_used  Repetition_counter=0  CH1_enable=on  CH1_type=Encoder  CH1_int=off  CH1_variable_duty=off  CH1_output_duty=[]  CH1_output_polarity=TIM_OCPolarity_High  CH1_output_comp_state=on  CH1_output_comp_polarity=TIM_OCNPolarity_High  CH1_output_idle=TIM_OCIdleState_Set  CH1_output_comp_idle=TIM_OCNIdleState_Set  CH1_input_polarity=TIM_ICPolarity_Rising  CH1_input_prescaler=TIM_ICPSC_DIV1  CH1_input_filter=0  CH1_input_it=No_interrupt  Encoder_TI1_polarity=TIM_ICPolarity_Rising  CH2_enable=on  CH2_type=Encoder  CH2_int=off  CH2_variable_duty=off  CH2_output_duty=[]  CH2_output_polarity=TIM_OCPolarity_High  CH2_output_comp_state=on  CH2_output_comp_polarity=TIM_OCNPolarity_High  CH2_output_idle=TIM_OCIdleState_Set  CH2_output_comp_idle=TIM_OCNIdleState_Set  CH2_input_polarity=TIM_ICPolarity_Rising  CH2_input_prescaler=TIM_ICPSC_DIV1  CH2_input_filter=0  CH2_input_it=No_interrupt  Encoder_TI2_polarity=TIM_ICPolarity_Rising  CH3_enable=off  CH3_type=Encoder  CH3_int=off  CH3_variable_duty=off  CH3_output_duty=[]  CH3_output_polarity=TIM_OCPolarity_High  CH3_output_comp_state=on  CH3_output_comp_polarity=TIM_OCNPolarity_High  CH3_output_idle=TIM_OCIdleState_Set  CH3_output_comp_idle=TIM_OCNIdleState_Set  CH3_input_polarity=TIM_ICPolarity_Rising  CH3_input_prescaler=TIM_ICPSC_DIV1  CH3_input_filter=0  CH3_input_it=No_interrupt
  USART_Config : USART_Lib/USART_Config  Commented=on  USART_CONFIG=USART3  USART_CONFIG_PIN=PC11/PC10 : (usart3 / uart4)  USART_SPEED=115200  USART_DATA=USART_WordLength_8b  USART_PARITY=USART_Parity_No  USART_STOP=USART_StopBits_1  USART_FLOW=off  USART_DEFAULT=off  It_rcv=on  It_send=on  Def_handler=on  Cust_handler=USART3_IRQHandler
  Unit Delay1 : UnitDelay  SampleTime=-1
  wires:
  MATLAB Function/2(Ib) -> Mux/2
  MATLAB Function/3(Ic) -> Mux/3
  Demux1/1 -> StartUp/1(DutyIn1)
  Demux1/2 -> StartUp/2(DutyIn2)
  Demux1/3 -> StartUp/3(DutyIn3)
  Encoder 2 Angle/1(Angle) -> Rate Transition2/1, AngleConv/1
  StartUp/1(Encoder_Reset) -> Timers1/1, Unit Delay1/1
  MATLAB Function/1(Ia) -> Mux/1
  StartUp/2(Duty1) -> Timers/1
  StartUp/4(Duty3) -> Timers/3
  Timers1/1 -> Encoder 2 Angle/1(Count)
  SVPWM/1(Duty) -> Demux1/1
  Saturation/1 -> SVPWM/1(Vabc)
  Speed Estimate/1(w) -> Rate Transition3/1
  Timers1/2 -> Rate Transition1/1
  Rate Transition1/1 -> Speed Estimate/2(Dir)
  Rate Transition2/1 -> Speed Estimate/1(Angle)
  StartUp/3(Duty2) -> Timers/2
  ADC_Read1/1 -> MATLAB Function/1(ADC1)
  ADC_Read1/2 -> MATLAB Function/2(ADC2)
  ADC_Read1/3 -> MATLAB Function/3(ADC3)
  Gain/1 -> Saturation/1
  ADC_Read/1 -> 0 to 1/2
  0 to 1/1 -> Add/1
  Add/1 -> Gain1/1
  Constant/1 -> Add/2
  Constant2/1 -> 0 to 1/1
  Unit Delay1/1 -> EncoderResetConv/1
  Gain1/1 -> Processing/2
  Mux/1 -> CurrentConv/1
  Processing/1 -> Gain/1
  EncoderResetConv/1 -> Processing/1
  AngleConv/1 -> Processing/4
  Rate Transition3/1 -> Processing/3
  CurrentConv/1 -> Processing/5

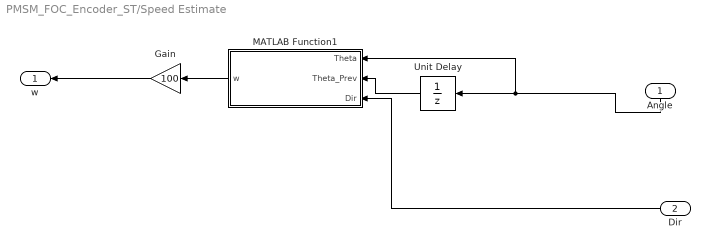
== system PMSM_FOC_Encoder_ST/Speed Estimate ==
  Angle : Inport
  Dir : Inport  Port=2
  Gain : Gain  Gain=100
  MATLAB Function1 : MATLAB Function  TreatAsAtomicUnit=on
  Unit Delay : UnitDelay  SampleTime=-1
  w : Outport
  wires:
  Unit Delay/1 -> MATLAB Function1/2(Theta_Prev)
  MATLAB Function1/1(w) -> Gain/1
  Angle/1 -> MATLAB Function1/1(Theta), Unit Delay/1
  Dir/1 -> MATLAB Function1/3(Dir)
  Gain/1 -> w/1

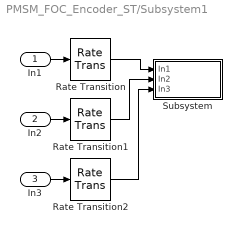
== system PMSM_FOC_Encoder_ST/Subsystem1 ==
  In1 : Inport
  In2 : Inport  Port=2
  In3 : Inport  Port=3
  Rate Transition : RateTransition
  Rate Transition1 : RateTransition
  Rate Transition2 : RateTransition
  Subsystem : Subsystem  TreatAsAtomicUnit=on  SystemSampleTime=0.05
      settings: MinAlgLoopOccurrences=on
  wires:
  Rate Transition2/1 -> Subsystem/3(In3)
  Rate Transition/1 -> Subsystem/1(In1)
  Rate Transition1/1 -> Subsystem/2(In2)
  In1/1 -> Rate Transition/1
  In3/1 -> Rate Transition2/1
  In2/1 -> Rate Transition1/1

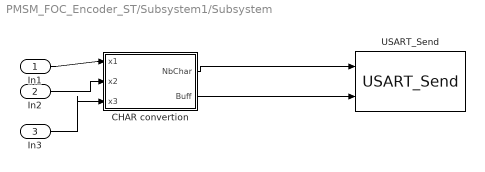
== system PMSM_FOC_Encoder_ST/Subsystem1/Subsystem ==
  In1 : Inport
  In2 : Inport  Port=2
  In3 : Inport  Port=3
  CHAR convertion : MATLAB Function  TreatAsAtomicUnit=on
  USART_Send : S-Function  FunctionName=USART_Send  Parameters=USART_name,NullString  EnableBusSupport=off  mask(USART_Send){USART_name=USART3, NullString=on}
      mask prompts: USART_name "Usart Name"; NullString "Null terminated string"
      mask help:
      | USART Send:
      | Send Nb2Send char on selected USART.
      | SendVal input must be a Null terminated array of char when "Null terminated string" parameter is selected.
      mask Help: web('help_USART_Send.html', '-helpbrowser')
      mask TypeOptions USART_name: USART1 | USART2 | USART3 | UART4 | UART5 | USART6
      mask Display:
      | color('blue'); text(0.6, 0.90, 'STM32F4xx', 'horizontalalignment', 'right');color('black'); text(0.50, 0.12, 'USART_Send', 'horizontalAlignment','center');
      | image(imread('ST.bmp','bmp'),'top-right');
      | port_label('input',1,'Nb2Send');
      | port_label('input',2,'SendVal');
      | port_label('output',1,'NbSent');
  wires:
  In1/1 -> CHAR convertion/1(x1)
  In2/1 -> CHAR convertion/2(x2)
  CHAR convertion/1(NbChar) -> USART_Send/1
  CHAR convertion/2(Buff) -> USART_Send/2
  In3/1 -> CHAR convertion/3(x3)

== stateflow chart PMSM_FOC_Encoder_ST/StartUp ==
  state Startup
    Encoder_Reset = 1;
    Duty1 = 30;
    Duty2 =-1;
    Duty3 = 5;
  state Running
    Encoder_Reset = 0;
    Duty1 = DutyIn1;
    Duty2 = DutyIn2;
    Duty3 = DutyIn3;
  (default) -> Startup
  Startup -> Running : [after(0.5,sec)]
  Running -> Running : [1]
  data: Encoder_Reset output int8 size=1; DutyIn1 input size=1; DutyIn2 input size=1; DutyIn3 input size=1; Duty1 output double size=1; Duty2 output double size=1; Duty3 output double size=1

== matlab function PMSM_FOC_Encoder_ST/Encoder 2 Angle ==
  data: Count input; Angle output; Params parameter
function Angle = Count2Angle(Count,Params)

Temp = cast(Count,'double');
Angle = (Temp*Params.Encoder_Gain+Params.Theta_Zero);
Angle = mod(Angle,2*pi);
end

== matlab function PMSM_FOC_Encoder_ST/MATLAB Function ==
  data: ADC1 input; ADC2 input; Ia output; ADC3 input; Ib output; Ic output
function [Ia,Ib,Ic] = Convert(ADC1,ADC2,ADC3)
% convert ADC output to amps (0.22 ohm resistors and gain of G=6.4)
% Vshunt = I*0.22*G 
% ADC out = Vshunt/3.3 * 4096
% I*0.22*G*4096/3.3
% I = ADC_out*3.3/0.22*G*4096

G = 6.4;
R = 0.22;
Offset = 1.94;
Va = ((cast(ADC1,'double')*3.3/4096)-Offset)/G;
Vb = ((cast(ADC2,'double')*3.3/4096)-Offset)/G;
Vc = ((cast(ADC3,'double')*3.3/4096)-Offset)/G;

Ia = -Va/R;
Ib = -Vb/R;
Ic = -Vc/R;

== matlab function PMSM_FOC_Encoder_ST/Subsystem1/Subsystem/CHAR convertion ==
  data: x1 input; NbChar output uint16 size=1; Buff output uint8 size=[1 20]; x2 input; x3 input
function [NbChar, Buff] = convert(x1,x2,x3)
u1 = cast(x1,'double');
u2 = cast(x2,'double');
u3 = cast(x3,'double');
%%Buff = uint32(0);
buffer1 = zeros(1,15,'uint8');
buffer2 = zeros(1,15,'uint8');
buffer3 = zeros(1,15,'uint8');
coder.ceval('sprintf',coder.wref(buffer1),['%2.2f',0],u1);
coder.ceval('sprintf',coder.wref(buffer2),['%2.2f',0],u2);
coder.ceval('sprintf',coder.wref(buffer3),['%2.2f',0],u3);
Buff = [uint8('x:'),buffer1(1:4), uint8('y:'),buffer2(1:4),uint8('z:'),buffer3(1:4),10, 0];
NbChar = uint16(size(Buff,2));

== matlab function PMSM_FOC_Encoder_ST/Speed Estimate/MATLAB Function1 ==
  data: Theta input; w output; Theta_Prev input; Dir input
function w = fcn(Theta,Theta_Prev,Dir)

% if Dir = 1 -> downcounting, Dir = 0 -> upcounting
if (Theta < Theta_Prev)&& (Dir == 0)
    % Positive Roll Over
    w = Theta+2*pi-Theta_Prev;
elseif (Theta > Theta_Prev)&& (Dir == 1)
    % Underflow
    w = Theta-2*pi-Theta_Prev;
else
    w = Theta-Theta_Prev;
end

== matlab function PMSM_FOC_Encoder_ST/SVPWM ==
  data: Vabc input; Duty output
function Duty = SVPWM(Vabc)

A = Vabc;
Duty = (A-ones(3,1)*(min(A)+max(A))*0.5)*2/sqrt(3);
Duty= ((Duty+1)/2)*100;
if (  Duty(1) < 0 )
    Duty(1) =0;
end;
if (  Duty(2) < 0 )
    Duty(2) =0;
end;
if (  Duty(3) < 0 )
    Duty(3) =0;
end;
if ( Duty(1) > 100)
    Duty(1) = 100;
end;
if ( Duty(2) > 100)
    Duty(2) = 100;
end;
if ( Duty(3) > 100)
    Duty(3) = 100;
end;
